simulink model "UDE_CT"  (R2020a)
settings: Solver=FixedStepAuto  StartTime=0.0  StopTime=tstop  FixedStep=tstep  RelTol=1e-3
values from neighbouring files (symbols this model uses):
  eic = xic - xmic    [data.m]
  Ts = 0.01    [data.m]
  udic = (-Ts/T)*(xtic(2) - xtmic(2))    [data.m]
  xic = [-3 2]'    [data.m]
  xmic = [1 1]'    [data.m]
settings Model: Creator=Maithili Shetty  LastModifiedBy=Ram Padmanabhan
settings DataIOCC: SaveOutput=off  SignalLogging=off  DSMLogging=off  SaveTime=off  ReturnWorkspaceOutputs=off

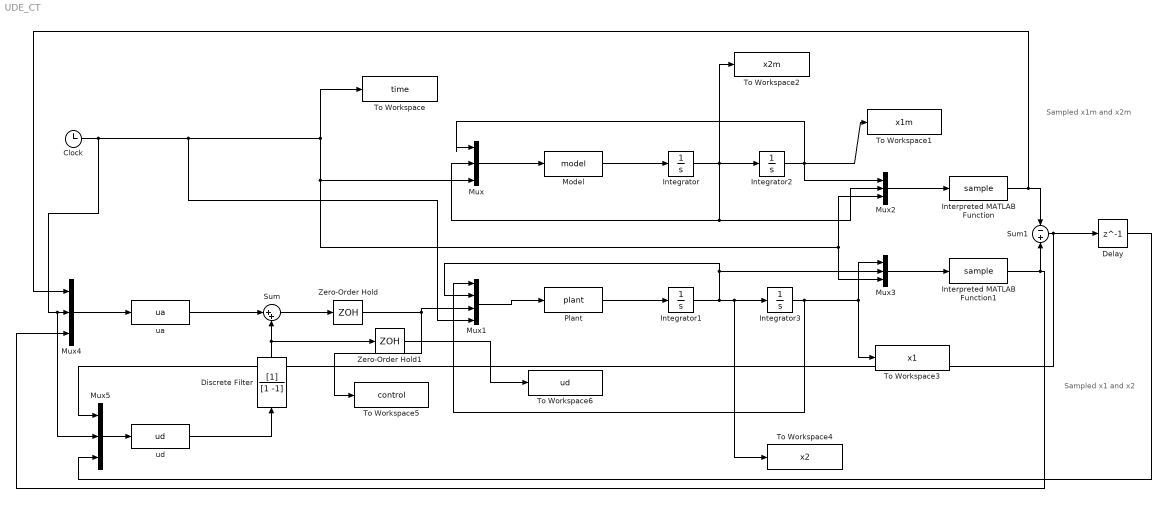
== system UDE_CT ==
  note: Sampled x1 and x2
  note: Sampled x1m and x2m
  Clock : Clock
  Delay : Delay  DelayLength=1  InitialCondition=eic  SampleTime=Ts
  Discrete Filter : DiscreteFilter  Denominator=[1 -1]  InitialStates=udic  SampleTime=Ts
  Integrator : Integrator  InitialCondition=xmic(2)
  Integrator1 : Integrator  InitialCondition=xic(2)
  Integrator2 : Integrator  InitialCondition=xmic(1)
  Integrator3 : Integrator  InitialCondition=xic(1)
  Interpreted MATLAB Function : MATLABFcn  MATLABFcn=sample  OutputDimensions=2
  Interpreted MATLAB Function1 : MATLABFcn  MATLABFcn=sample  OutputDimensions=2
  Model : MATLABFcn  MATLABFcn=model  OutputDimensions=1
  Mux{,2..5} (5 alike) : Mux  Inputs=3
  Mux1 : Mux
  Plant : MATLABFcn  MATLABFcn=plant  OutputDimensions=1
  Sum : Sum  Inputs=|++
  Sum1 : Sum  Inputs=-+
  To Workspace : ToWorkspace  VariableName=time  SampleTime=-1
  To Workspace1 : ToWorkspace  VariableName=x1m  SampleTime=-1
  To Workspace2 : ToWorkspace  VariableName=x2m  SampleTime=-1
  To Workspace3 : ToWorkspace  VariableName=x1  SampleTime=-1
  To Workspace4 : ToWorkspace  VariableName=x2  SampleTime=-1
  To Workspace5 : ToWorkspace  VariableName=control  SampleTime=-1
  To Workspace6 : ToWorkspace  VariableName=ud  SampleTime=-1
  Zero-Order Hold : ZeroOrderHold  SampleTime=Ts
  Zero-Order Hold1 : ZeroOrderHold  SampleTime=Ts
  ua : MATLABFcn  MATLABFcn=ua  OutputDimensions=1
  ud : MATLABFcn  MATLABFcn=ud  OutputDimensions=1
  wires:
  Model/1 -> Integrator/1
  Plant/1 -> Integrator1/1
  Integrator/1 -> Mux2/2, Mux/2, Integrator2/1, To Workspace2/1
  Integrator1/1 -> Mux1/2, Mux3/2, To Workspace4/1, Integrator3/1
  Integrator2/1 -> Mux/1, To Workspace1/1, Mux2/1
  Mux/1 -> Model/1
  Clock/1 -> Mux1/4, Mux3/3, Mux2/3, Mux/3, To Workspace/1, Mux5/2, Mux4/2
  Integrator3/1 -> Mux1/1, To Workspace3/1, Mux3/1
  Mux1/1 -> Plant/1
  Mux2/1 -> Interpreted MATLAB Function/1
  Mux3/1 -> Interpreted MATLAB Function1/1
  Interpreted MATLAB Function/1 -> Sum1/1, Mux4/1
  Interpreted MATLAB Function1/1 -> Mux4/3, Sum1/2
  Zero-Order Hold/1 -> To Workspace5/1, Mux1/3
  ud/1 -> Discrete Filter/1
  ua/1 -> Sum/1
  Discrete Filter/1 -> Sum/2, Zero-Order Hold1/1
  Sum/1 -> Zero-Order Hold/1
  Mux4/1 -> ua/1
  Zero-Order Hold1/1 -> To Workspace6/1
  Sum1/1 -> Mux5/1, Delay/1
  Mux5/1 -> ud/1
  Delay/1 -> Mux5/3
